simulink model "NonlinearModel_NonlinearController"  (R2017b)
settings: Solver=ode4  StartTime=0.0  StopTime=time  FixedStep=step_size  RelTol=1e-3  EnableMultiTasking=on
values from neighbouring files (symbols this model uses):
  angle_restrict = pi/1.5    (= 2.09439510239)    [NonLinearAnimations.m]    (also in experiment_vs_simulated.m)
  Kd = 12.7    [NonLinearAnimations.m]    (also in experiment_vs_simulated.m; vars_for_mcu.m)
  Kp = 58    [NonLinearAnimations.m]    (also in experiment_vs_simulated.m; vars_for_mcu.m)
  motor_stall_torque = 6    [LinearAnimations.m]    (also in LinearisedModel.m = 2.8; NonLinearAnimations.m = 8; experiment_vs_simulated.m = 8)
  phi_dot_start = 0    [LinearAnimations.m]    (also in NonLinearAnimations.m; experiment_vs_simulated.m)
  phi_start = -pi/20    (= -0.157079632679)    [LinearAnimations.m]    (also in NonLinearAnimations.m = 0; experiment_vs_simulated.m = -1.502)
  region_1 = pi/50    (= 0.0628318530718)    [NonLinearAnimations.m]    (also in experiment_vs_simulated.m)
  region_2 = pi/5    (= 0.628318530718)    [NonLinearAnimations.m]    (also in experiment_vs_simulated.m)
  theta_dot_start = 0    [LinearAnimations.m]    (also in NonLinearAnimations.m; experiment_vs_simulated.m)
  theta_start = pi+pi/50    (= 3.20442450666)    [LinearAnimations.m]    (also in NonLinearAnimations.m = 0.10471975512; experiment_vs_simulated.m = 0)
settings Model: Creator=Henry  LastModifiedBy=Henry
settings SolverCC: NumberNewtonIterations=5  MaxConsecutiveMinStep=2
settings DataIOCC: SaveState=on
settings OptimizationCC: UseFloatMulNetSlope=on
settings CodeAppCC: StateflowObjectComments=on

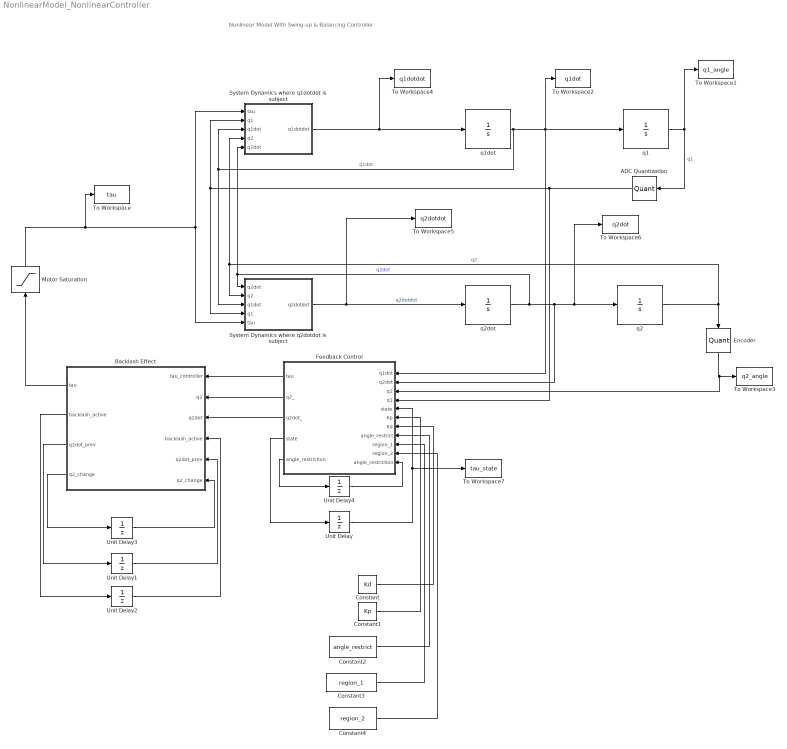
== system NonlinearModel_NonlinearController ==
  note: Nonlinear Model With Swing-up & Balancing Controller
  ADC Quantization : Quantizer  QuantizationInterval=ADC_resolution  LinearizeAsGain=off
  Backlash Effect : MATLAB Function  TreatAsAtomicUnit=on
  Constant : Constant  Value=Kd
  Constant1 : Constant  Value=Kp
  Constant2 : Constant  Value=angle_restrict
  Constant3 : Constant  Value=region_1
  Constant4 : Constant  Value=region_2
  Encoder : Quantizer  QuantizationInterval=encoder_resolution  LinearizeAsGain=off
  "Feedback Control " : MATLAB Function  TreatAsAtomicUnit=on
  Motor Saturation : Saturate  UpperLimit=motor_stall_torque  LowerLimit=-1*motor_stall_torque
  System Dynamics where q2dotdot is subject : MATLAB Function  TreatAsAtomicUnit=on
  System Dynamics where q1dotdot is subject : MATLAB Function  TreatAsAtomicUnit=on
  To Workspace : ToWorkspace  VariableName=tau  SaveFormat=Timeseries  SampleTime=-1
  To Workspace1 : ToWorkspace  VariableName=q1_angle  SaveFormat=Timeseries  SampleTime=-1
  To Workspace2 : ToWorkspace  VariableName=q1dot  SaveFormat=Timeseries  SampleTime=-1
  To Workspace3 : ToWorkspace  VariableName=q2_angle  SaveFormat=Timeseries  SampleTime=-1
  To Workspace4 : ToWorkspace  VariableName=q1dotdot  SaveFormat=Timeseries  SampleTime=-1
  To Workspace5 : ToWorkspace  VariableName=q2dotdot  SaveFormat=Timeseries  SampleTime=-1
  To Workspace6 : ToWorkspace  VariableName=q2dot  SaveFormat=Timeseries  SampleTime=-1
  To Workspace7 : ToWorkspace  VariableName=tau_state  SaveFormat=Timeseries  SampleTime=-1
  Unit Delay{,1..4} (5 alike) : UnitDelay  SampleTime=-1
  q1 : Integrator  InitialCondition=theta_start  ContinuousStateAttributes='angle_q1'
  q1dot : Integrator  InitialCondition=theta_dot_start
  q2 : Integrator  InitialCondition=phi_start  ContinuousStateAttributes='angle_2'
  q2dot : Integrator  InitialCondition=phi_dot_start
  wires:
  q1dot/1 -> System Dynamics where q2dotdot is subject/3(q1dot), System Dynamics where q1dotdot is subject/3(q1dot), To Workspace2/1, "Feedback Control "/1(q1dot), q1/1  "q1dot"
  System Dynamics where q1dotdot is subject/1(q1dotdot) -> q1dot/1, To Workspace4/1
  System Dynamics where q2dotdot is subject/1(q2dotdot) -> q2dot/1, To Workspace5/1  "q2dotdot"
  q2dot/1 -> System Dynamics where q2dotdot is subject/1(q2dot), System Dynamics where q1dotdot is subject/5(q2dot), To Workspace6/1, q2/1, "Feedback Control "/2(q2dot)  "q2dot"
  q2/1 -> System Dynamics where q1dotdot is subject/4(q2), System Dynamics where q2dotdot is subject/2(q2), Encoder/1  "q2"
  q1/1 -> ADC Quantization/1, To Workspace1/1  "q1"
  "Feedback Control "/1(tau) -> Backlash Effect/1(tau_controller)
  Motor Saturation/1 -> System Dynamics where q1dotdot is subject/1(tau), System Dynamics where q2dotdot is subject/5(tau), To Workspace/1
  "Feedback Control "/4(state) -> Unit Delay/1
  Unit Delay/1 -> To Workspace7/1, "Feedback Control "/5("state ")
  Constant1/1 -> "Feedback Control "/6(Kp)
  Constant/1 -> "Feedback Control "/7(Kd)
  Constant2/1 -> "Feedback Control "/8(angle_restrict)
  Constant3/1 -> "Feedback Control "/9(region_1)
  Constant4/1 -> "Feedback Control "/10(region_2)
  Backlash Effect/1(tau) -> Motor Saturation/1
  Encoder/1 -> "Feedback Control "/3(q2), To Workspace3/1
  ADC Quantization/1 -> System Dynamics where q1dotdot is subject/2(q1), System Dynamics where q2dotdot is subject/4(q1), "Feedback Control "/4(q1)
  Backlash Effect/3(q2dot_prev) -> Unit Delay1/1
  Backlash Effect/2(backlash_active) -> Unit Delay2/1
  Unit Delay1/1 -> Backlash Effect/5("q2dot_prev ")
  Unit Delay2/1 -> Backlash Effect/4("backlash_active ")
  "Feedback Control "/2(q2_) -> Backlash Effect/2(q2)
  "Feedback Control "/3(q2dot_) -> Backlash Effect/3(q2dot)
  Backlash Effect/4(q2_change) -> Unit Delay3/1
  Unit Delay3/1 -> Backlash Effect/6("q2_change ")
  "Feedback Control "/5(angle_restriction) -> Unit Delay4/1
  Unit Delay4/1 -> "Feedback Control "/11("angle_restriction ")

== matlab function NonlinearModel_NonlinearController/System Dynamics where q2dotdot is subject ==
  data: q2dot input; q2 input; q1dot input; q1 input; tau input; q2dotdot output
function q2dotdot = fcn(q2dot, q2, q1dot,q1, tau)
%% System Constants
g = 9.81;
Ia = 0.0024;
Ib = 0.0035;
L1 = 0.2350;
L2 = 0.2600;
l1 = 0.2250;
l2 = 0.2350;
m1 = 0.5763;
m2 = 0.49277;
f1 = 6.6590e-04;
f2 = 0.0030;

%% System Dynamics
A = m1*l1^2 + m2*L1^2 + m2*l2^2 + 2*m2*l2*L1*cos(q2) + Ia + Ib;
B = m2*l2^2 + m2*L1*l2*cos(q2) + Ib;
E = m1*g*l1*sin(q1);
F = m2*g*L1*sin(q1);
G = m2*g*l2*sin(q1+q2);
C = 2*m2*l2*L1*q1dot*q2dot*sin(q2);
D = m2*L1*l2*q2dot^2*sin(q2);

H = m2*l2^2 + m2*L1*l2*cos(q2) + Ib;
I = m2*l2^2 + Ib ;
K = m2*L1*l2*q1dot^2*sin(q2);
J  = m2*L1*l2*q1dot*q2dot*sin(q2);
M = m2*g*l2*sin(q1+q2);
L  = m2*L1*l2*q1dot*q2dot*sin(q2);
% Coefficient for Damping 

Z = -f1*q1dot;
Y = -f2*(q2dot-q1dot)+tau;

alpha = -C-D+E+F+G-Z;
zeta = -J+K+L+M-Y;

AA = [A,B;H,I];
BB = [-alpha;-zeta];

meep = AA\BB;
q2dotdot = meep(end,1);

== matlab function NonlinearModel_NonlinearController/System Dynamics where q1dotdot is subject ==
  data: tau input; q1 input; q1dot input; q2 input; q2dot input; q1dotdot output
function q1dotdot = fcn(tau, q1, q1dot,q2, q2dot)
%% System Constants
g = 9.81;
Ia = 0.0024;
Ib = 0.0035;
L1 = 0.2350;
L2 = 0.2600;
l1 = 0.2250;
l2 = 0.2350;
m1 = 0.5763;
m2 = 0.49277;
f1 = 6.6590e-04;
f2 = 0.0030;


%% Dynamics
A = m1*l1^2 + m2*L1^2 + m2*l2^2 + 2*m2*l2*L1*cos(q2) + Ia + Ib;
B = m2*l2^2 + m2*L1*l2*cos(q2) + Ib;
E = m1*g*l1*sin(q1);
F = m2*g*L1*sin(q1);
G = m2*g*l2*sin(q1+q2);
C = 2*m2*l2*L1*q1dot*q2dot*sin(q2);
D = m2*L1*l2*q2dot^2*sin(q2);

H = Ib+m2*l2^2+m2*L1*l2*cos(q2);
I = Ib+m2*l2^2;
K = m2*L1*l2*q1dot^2*sin(q2);
J = m2*L1*l2*q1dot*q2dot*sin(q2);
M = m2*g*l2*sin(q1+q2);
L = m2*L1*l2*q1dot*q2dot*sin(q2);
% Coefficient for Damping 
Z = -f1*q1dot;
Y = -f2*(q2dot-q1dot)+tau;

alpha = -C-D+E+F+G-Z;
zeta = -J+K+L+M-Y;

AA = [A,B;H,I];
BB = [-alpha;-zeta];

meep = AA\BB;
q1dotdot = meep(1,1);

== matlab function NonlinearModel_NonlinearController/Feedback Control  ==
  data: q1dot input; q2dot input; tau output; q2_ output; q2dot_ output; q2 input; q1 input; state input; state output; Kp input; Kd input; angle_restrict input; region_1 input; region_2 input; angle_restriction output; angle_restriction input
function [tau,q2_,q2dot_,state,angle_restriction]= feedback_control( q1dot, q2dot, q2, q1,state,Kp,Kd,angle_restrict,region_1,region_2, angle_restriction)
%% Pass variables through
q2_ = q2;
q2dot_ = q2dot;


%% System Constants
g = 9.81;
Ia = 0.0265152541;
Ib = 0.0221429705;
L1 = 0.2350;
L2 = 0.245;
l1 = 0.235;
l2 = 0.245;
m1 = 0.5763;
m2 = 0.49277;
f1 = 1.0953e-04;
f2 = 0.0028;


A = Ia+Ib+m1*l2^2+m2*L1^2+m2*l2^2+2*m2*l2*L1*cos(q2);
B = Ib+m2*l2^2+m2*L1*l2*cos(q2);
E = m1*g*l1*sin(q1);
F = m2*g*L1*sin(q1);
G = m2*g*l2*sin(q1+q2);
C = 2*m2*l2*L1*q1dot*q2dot*sin(q2);
D = m2*L1*l2*q2dot^2*sin(q2);

H =Ib+m2*l2^2+m2*L1*l2*cos(q2);
I =Ib+m2*l2^2;
K = m2*L1*l2*q1dot^2*sin(q2);
J = m2*L1*l2*q1dot*q2dot*sin(q2);
M = m2*g*l2*sin(q1+q2);
L = m2*L1*l2*q1dot*q2dot*sin(q2);
% Coefficient for Damping 

Z = -f1*q1dot;
Y = -f2*(q2dot-q1dot);

%% Collocated Linearization
alpha = -C-D+E+F+G-Z;
zeta = -J+K+L+M-Y;

v2 = 5*(20*(pi/0.9*atan(q1dot)-q2)-8*q2dot);
tau = 0; 

    if( ( q1 > pi*0.3 || q1 < -pi*0.3) && state == 0)
        state = 1;
        angle_restriction = pi/70;    
    end

    if( ( q1 > pi*0.95 || q1 < -pi*0.95  ) && state == 1)
        state = 2;
        angle_restriction = pi/70;
        
    end
    
    if( ( q1 > (pi-region_1) || q1 < (-pi+region_1) ) && (q2 < region_2 && q2 > -region_2) && state == 2)
        state = 4;
    end
    
    if(  state == 4)
        K = [-24.9855   -8.1096   -5.1358   -2.2153];
       tau = -K*[q1-pi;q2;q1dot;q2dot];
%        tau = 0;
       
    elseif(state == 1)
        v2 = 1*(Kp*(angle_restriction*atan(q1dot)-q2)-Kd*q2dot);
        tau = zeta - H*alpha/A + (I-B*H/A)*v2;

    elseif(state == 2)
        v2 = (Kp*(angle_restriction*atan(q1dot)-q2)-Kd*q2dot);
        tau = zeta - H*alpha/A + (I-B*H/A)*v2;        
        
    elseif( state == 0)
        v2 = 1*(Kp*(angle_restrict*atan(q1dot)-q2)-Kd*q2dot);
        tau = zeta - H*alpha/A + (I-B*H/A)*v2;
    end
    
 %% Verification Test:

== matlab function NonlinearModel_NonlinearController/Backlash Effect ==
  data: tau_controller input; q2 input; q2dot input; tau output; backlash_active input; q2dot_prev input; backlash_active output; q2dot_prev output; q2_change input; q2_change output
function [tau,backlash_active,q2dot_prev,q2_change] = gearbox_backlash(tau_controller,q2,q2dot,backlash_active,q2dot_prev,q2_change)

tau = tau_controller;
% backlash_constant = 0.0175;    % [rad]
% 
% if (q2dot > 0 && q2dot_prev < 0)
%     backlash_active = 1;
%     q2_change = q2;
%     tau = 0;
% end
% 
% if (q2dot < 0 && q2dot_prev > 0)
%     backlash_active = -1;
%     q2_change = q2;
%     tau = 0;
% end
% 
% if ( (backlash_active == -1 && q2 > (q2_change + backlash_active*backlash_constant)) || (backlash_active == 1 && q2 < (q2_change + backlash_active*backlash_constant)) )
%     tau = 0;
% else
%     backlash_active = 0;
%     tau = tau_controller;
%     
% end
% q2dot_prev = q2dot;
% tau = tau_controller;
